simulink model "revised_model"  (R2017a)
settings: Solver=FixedStepAuto  StartTime=0.0  StopTime=60  FixedStep=0.001  RelTol=1e-3
values from neighbouring files (symbols this model uses):
  A = 0    [model_parameter.m]
  a = 0.4    [model_parameter.m]
  a_d = a * negative_gain    (= 0.38)    [model_parameter.m]
  alpha1 = 0.5    [model_parameter.m]
  alpha2 = 0.25    [model_parameter.m]
  B = 1    [model_parameter.m]
  b = 0.4    [model_parameter.m]
  b_d = b * positive_gain    (= 0.42)    [model_parameter.m]
  beta1 = 100    [model_parameter.m]
  beta2 = 300    [model_parameter.m]
  beta3 = 1000    [model_parameter.m]
  C = 1    [model_parameter.m]
  cl = c    (= 0.271)    [model_parameter.m]
  cl_d = c * negative_gain    (= 0.25745)    [model_parameter.m]
  cr = c    (= 0.271)    [model_parameter.m]
  cr_d = c * positive_gain    (= 0.28455)    [model_parameter.m]
  D = 0    [model_parameter.m]
  delta = 0.002    [model_parameter.m]
  k1 = 5    [model_parameter.m]
  k2 = 8    [model_parameter.m]
  k3 = 8    [model_parameter.m]
  k4 = [35 35]    [model_parameter.m]
  k5 = 0    [model_parameter.m]
  k6 = [0.1 0.1]    [model_parameter.m]
  kp = 0.2    [model_parameter.m]
  M = [m 0 0; 0 m 0; 0 0 I]    [model_parameter.m]
  m = 20    [model_parameter.m]
  M_d = [m_d 0 0; 0 m_d 0; 0 0 I_d]    [model_parameter.m]
  m_d = m * positive_gain    (= 21)    [model_parameter.m]
  r = 0.112    [model_parameter.m]
  r_d = r * negative_gain    (= 0.1064)    [model_parameter.m]
  Ts = 0.01    [model_parameter.m]
  ux = 0.02    [model_parameter.m]
  uy = 0.1    [model_parameter.m]
  XICR = 0    [model_parameter.m]
  XICR_d = XICR    (= 0)    [model_parameter.m]
undefined symbols (not defined in the file or in its folder): Continuous, DiscIntNeverNeededParam, Time
libraries: simulink x18, ctrlSharedLib x1
settings Model: Creator=Totorowithme  LastModifiedBy=Totorowithme
settings OptimizationCC: LifeSpan=inf
settings DebuggingCC: SFExecutionAtInitializationDiag=none

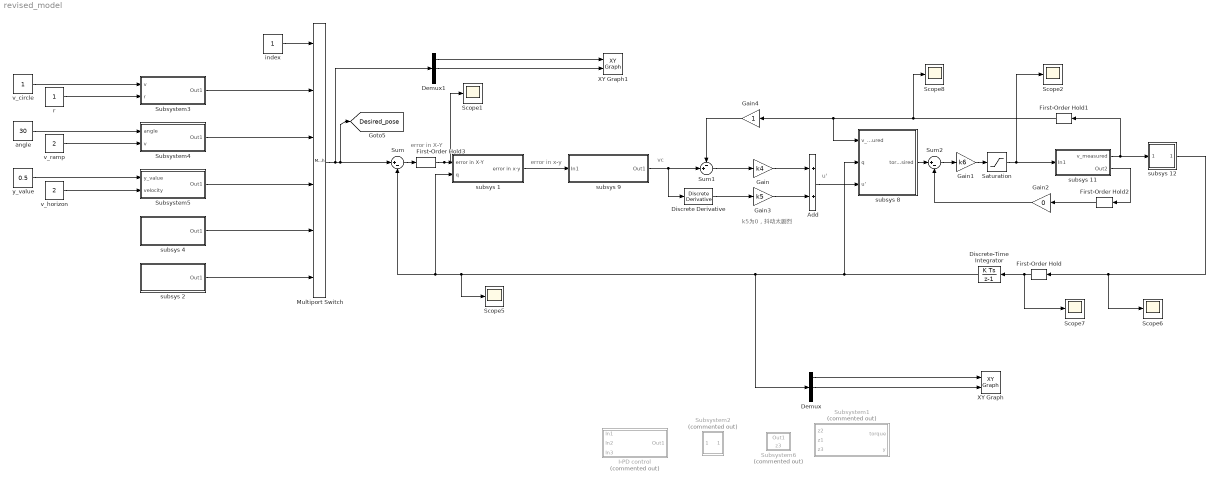
== system revised_model ==
  note: k5为0，抖动太剧烈
  note: u'
  note: vc
  note: error in x-y
  note: error in X-Y
  Add : Sum
  Demux : Demux  Outputs=3
  Demux1 : Demux  Outputs=3
  Discrete Derivative : simulink/Discrete/Discrete Derivative  gainval=1.0  ICPrevScaledInput=0.0  OutMin=[]  OutMax=[]  OutDataType=fixdt(1, 16)  OutScaling=2^-10  DoSatur=off
  Discrete-Time Integrator : DiscreteIntegrator  InitialConditionSetting=State (most efficient)  SampleTime=0.01  ICPrevOutput=DiscIntNeverNeededParam  ICPrevScaledInput=DiscIntNeverNeededParam
  First-Order Hold{,1..3} (4 alike) : simulink/Discrete/First-Order Hold  DisableCoverage=on  Ts=0.01
      settings: SourceProductName=Simulink  SourceProductBaseCode=SL
  Gain : Gain  Gain=k4
  Gain1 : Gain  Gain=k6
  Gain2 : Gain  Gain=0
  Gain3 : Gain  Gain=k5
  Gain4 : Gain
  I-PD control : Subsystem  Commented=on
  Multiport Switch : MultiPortSwitch  Inputs=5
  Saturation : Saturate  UpperLimit=3  LowerLimit=-3
  Scope{1..2,5..8} (6 alike) : Scope
  Subsystem1 : Subsystem  Commented=on
      mask Display: disp('Extended state observer','texmode','on')
  Subsystem2 : Subsystem  Commented=on
      mask Display: disp('inv(S)', 'texmode', 'on')
  Subsystem3 : Subsystem
      mask Display: disp('circle','texmode','on')
  Subsystem4 : Subsystem
      mask Display: disp('ramp','texmode','on')
  Subsystem5 : Subsystem
      mask Display: disp('horizontal line','texmode','on')
  Subsystem6 : Subsystem  Commented=on
      mask Display: disp('inv(H)', 'texmode', 'on')
  Sum : Sum  Inputs=|+-
  Sum1 : Sum  Inputs=-+|
  Sum2 : Sum  Inputs=|+-
  XY Graph : simulink/Sinks/XY Graph  xmin=-12  xmax=12  ymin=-12  ymax=12  st=-1
  XY Graph1 : simulink/Sinks/XY Graph  xmin=-12  xmax=12  ymin=-12  ymax=12  st=-1
  angle : Constant  Value=30
  index : Constant
  r : Constant
  subsys 1 : Subsystem
      mask Display: disp('Transfer from X-Y to x-y','texmode','on')
  subsys 11 : Subsystem
      mask Display: disp('Dynamic function','texmode','on')
  subsys 12 : Subsystem
      mask Display: disp('S(q)','texmode','on')
  subsys 2 : Subsystem
      mask Display: disp('Desired pose','texmode','on')
  subsys 4 : Subsystem
      mask Display: disp('Desired pose','texmode','on')
  subsys 8 : Subsystem
      mask Display: disp('Torque control','texmode','on')
  subsys 9 : Subsystem
      mask Display: disp('Auxiliary velocity control','texmode','on')
  v_circle : Constant
  v_horizon : Constant  Value=2
  v_ramp : Constant  Value=2
  y_value : Constant  Value=0.5
  tag scope: Desired_pose=global
  wires:
  v_circle/1 -> Subsystem3/1(v)
  Subsystem3/1(Out1) -> Multiport Switch/2
  subsys 2/1(Out1) -> Multiport Switch/6
  Subsystem5/1(Out1) -> Multiport Switch/4
  Subsystem4/1(Out1) -> Multiport Switch/3
  r/1 -> Subsystem3/2(r)
  angle/1 -> Subsystem4/1(angle)
  index/1 -> Multiport Switch/1
  v_ramp/1 -> Subsystem4/2(v)
  v_horizon/1 -> Subsystem5/2(velocity)
  subsys 4/1(Out1) -> Multiport Switch/5
  y_value/1 -> Subsystem5/1(y_value)
  Sum/1 -> First-Order Hold3/1
  subsys 1/1(error in x-y) -> subsys 9/1(In1)
  subsys 9/1(Out1) -> Sum1/2, Discrete Derivative/1
  Sum1/1 -> Gain/1
  subsys 12/1(Out1) -> Scope6/1, First-Order Hold/1
  Discrete-Time Integrator/1 -> subsys 8/2(q), Demux/1, Scope5/1, subsys 1/2(q), Sum/2
  Demux/1 -> XY Graph/1
  Demux/2 -> XY Graph/2
  Add/1 -> subsys 8/3(u')
  subsys 11/2(Out2) -> First-Order Hold2/1
  subsys 8/1(torque_desired) -> Sum2/1
  Sum2/1 -> Gain1/1
  Gain1/1 -> Saturation/1
  Discrete Derivative/1 -> Gain3/1
  Gain3/1 -> Add/2
  First-Order Hold/1 -> Discrete-Time Integrator/1, Scope7/1
  First-Order Hold3/1 -> Scope1/1, subsys 1/1(error in X-Y)
  subsys 11/1(v_measured) -> subsys 12/1(In1), First-Order Hold1/1
  Gain4/1 -> Sum1/1
  First-Order Hold2/1 -> Gain2/1
  Gain2/1 -> Sum2/2
  Saturation/1 -> subsys 11/1(In1), Scope2/1
  First-Order Hold1/1 -> Gain4/1, subsys 8/1(v_measured), Scope8/1
  Gain/1 -> Add/1
  Demux1/2 -> XY Graph1/2
  Demux1/1 -> XY Graph1/1
  Multiport Switch/1 -> Sum/1, [Desired_pose], Demux1/1

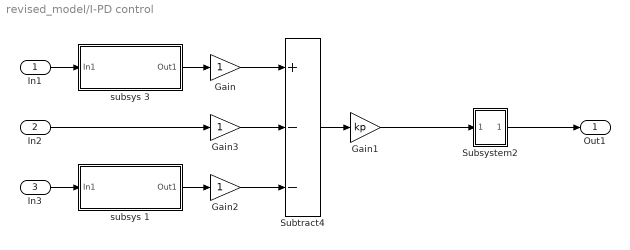
== system revised_model/I-PD control ==
  In1 : Inport
  In2 : Inport  Port=2
  In3 : Inport  Port=3
  Gain : Gain
  Gain1 : Gain  Gain=kp
  Gain2 : Gain
  Gain3 : Gain
  Subsystem2 : Subsystem
      mask Display: disp('inv(S)', 'texmode', 'on')
  Subtract4 : Sum  Inputs=+--
  subsys 1 : Subsystem
      mask Display: disp('transfer2','texmode','on')
  subsys 3 : Subsystem
      mask Display: disp('transfer1','texmode','on')
  Out1 : Outport
  wires:
  In1/1 -> subsys 3/1(In1)
  In3/1 -> subsys 1/1(In1)
  In2/1 -> Gain3/1
  subsys 1/1(Out1) -> Gain2/1
  Subtract4/1 -> Gain1/1
  Gain1/1 -> Subsystem2/1(dq)
  Subsystem2/1(Out1) -> Out1/1
  subsys 3/1(Out1) -> Gain/1
  Gain/1 -> Subtract4/1
  Gain2/1 -> Subtract4/3
  Gain3/1 -> Subtract4/2

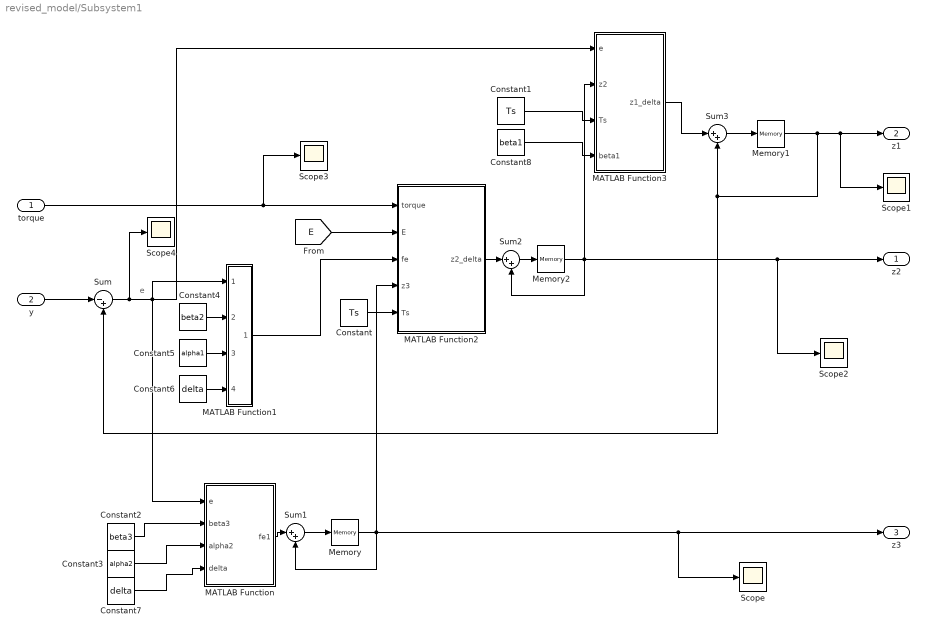
== system revised_model/Subsystem1 ==
  note: e
  torque : Inport
  y : Inport  Port=2
  Constant : Constant  Value=Ts
  Constant1 : Constant  Value=Ts
  Constant2 : Constant  Value=beta3
  Constant3 : Constant  Value=alpha2
  Constant4 : Constant  Value=beta2
  Constant5 : Constant  Value=alpha1
  Constant6 : Constant  Value=delta
  Constant7 : Constant  Value=delta
  Constant8 : Constant  Value=beta1
  MATLAB Function : MATLAB Function  TreatAsAtomicUnit=on
  MATLAB Function1 : MATLAB Function  TreatAsAtomicUnit=on
  MATLAB Function2 : MATLAB Function  TreatAsAtomicUnit=on
  MATLAB Function3 : MATLAB Function  TreatAsAtomicUnit=on
  Memory : Memory  X0=[0 0 0]
  Memory1 : Memory  X0=[0 0 0]
  Memory2 : Memory  X0=[0 0 0]
  Scope{,1..4} (5 alike) : Scope
  Sum : Sum  Inputs=|-+
  Sum1 : Sum  Inputs=|++
  Sum2 : Sum  Inputs=|++
  Sum3 : Sum  Inputs=|++
  z2 : Outport
  z1 : Outport  Port=2
  z3 : Outport  Port=3
  wires:
  y/1 -> Sum/1
  Sum/1 -> Scope4/1, MATLAB Function1/1(e), MATLAB Function3/1(e), MATLAB Function/1(e)
  Sum1/1 -> Memory/1
  MATLAB Function/1(fe1) -> Sum1/1
  MATLAB Function1/1(fe) -> MATLAB Function2/3(fe)
  [E] -> MATLAB Function2/2(E)
  torque/1 -> Scope3/1, MATLAB Function2/1(torque)
  MATLAB Function2/1(z2_delta) -> Sum2/1
  MATLAB Function3/1(z1_delta) -> Sum3/1
  Constant/1 -> MATLAB Function2/5(Ts)
  Constant1/1 -> MATLAB Function3/3(Ts)
  Constant2/1 -> MATLAB Function/2(beta3)
  Constant3/1 -> MATLAB Function/3(alpha2)
  Constant4/1 -> MATLAB Function1/2(beta2)
  Constant5/1 -> MATLAB Function1/3(alpha1)
  Constant6/1 -> MATLAB Function1/4(delta)
  Constant7/1 -> MATLAB Function/4(delta)
  Constant8/1 -> MATLAB Function3/4(beta1)
  Sum2/1 -> Memory2/1
  Sum3/1 -> Memory1/1
  Memory/1 -> Sum1/2, Scope/1, z3/1, MATLAB Function2/4(z3)
  Memory2/1 -> Scope2/1, z2/1, Sum2/2, MATLAB Function3/2(z2)
  Memory1/1 -> Scope1/1, z1/1, Sum3/2, Sum/2

== system revised_model/Subsystem2 ==
  dq : Inport
  MATLAB Function : MATLAB Function  TreatAsAtomicUnit=on
  Out1 : Outport
  wires:
  [S] -> MATLAB Function/1(S)
  dq/1 -> MATLAB Function/2(dq)
  MATLAB Function/1(v) -> Out1/1

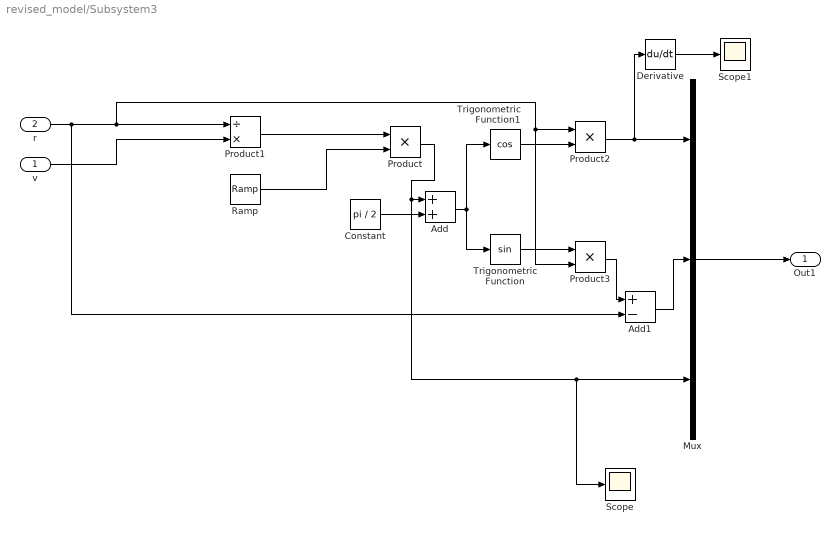
== system revised_model/Subsystem3 ==
  v : Inport
  r : Inport  Port=2
  Add : Sum
  Add1 : Sum  Inputs=+-
  Constant : Constant  Value=pi / 2
  Derivative : Derivative
  Mux : Mux  Inputs=3
  Product : Product
  Product1 : Product  Inputs=/*
  Product2 : Product
  Product3 : Product
  Ramp : simulink/Sources/Ramp  slope=-1  start=0  X0=0
  Scope : Scope
  Scope1 : Scope
  Trigonometric Function : Trigonometry
  Trigonometric Function1 : Trigonometry  Operator=cos
  Out1 : Outport
  wires:
  v/1 -> Product1/2
  r/1 -> Add1/2, Product3/2, Product2/1, Product1/1
  Product1/1 -> Product/1
  Trigonometric Function1/1 -> Product2/2
  Trigonometric Function/1 -> Product3/1
  Product2/1 -> Derivative/1, Mux/1
  Product/1 -> Scope/1, Mux/3, Add/1
  Constant/1 -> Add/2
  Add/1 -> Trigonometric Function/1, Trigonometric Function1/1
  Product3/1 -> Add1/1
  Add1/1 -> Mux/2
  Ramp/1 -> Product/2
  Mux/1 -> Out1/1
  Derivative/1 -> Scope1/1

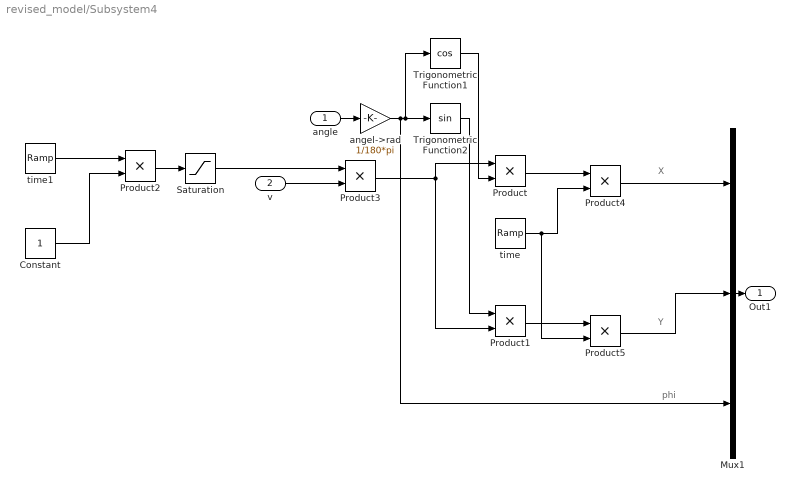
== system revised_model/Subsystem4 ==
  note: phi
  note: Y
  note: X
  angle : Inport
  v : Inport  Port=2
  Constant : Constant
  Mux1 : Mux  Inputs=3
  Product{,1..5} (6 alike) : Product
  Saturation : Saturate  UpperLimit=1  LowerLimit=0
  Trigonometric Function1 : Trigonometry  Operator=cos
  Trigonometric Function2 : Trigonometry
  angel->rad : Gain  Gain=1/180*pi
  time : simulink/Sources/Ramp  slope=1  start=0  X0=0
  time1 : simulink/Sources/Ramp  slope=1  start=0  X0=0
  Out1 : Outport
  wires:
  angle/1 -> angel->rad/1
  Trigonometric Function1/1 -> Product/2
  angel->rad/1 -> Mux1/3, Trigonometric Function1/1, Trigonometric Function2/1
  Trigonometric Function2/1 -> Product1/1
  Product/1 -> Product4/1
  time/1 -> Product5/2, Product4/2
  Product1/1 -> Product5/1
  Product4/1 -> Mux1/1
  Mux1/1 -> Out1/1
  Product5/1 -> Mux1/2
  time1/1 -> Product2/1
  Constant/1 -> Product2/2
  Saturation/1 -> Product3/1
  v/1 -> Product3/2
  Product2/1 -> Saturation/1
  Product3/1 -> Product1/2, Product/1

== system revised_model/Subsystem5 ==
  y_value : Inport
  velocity : Inport  Port=2
  Constant2 : Constant  Value=0
  Mux1 : Mux  Inputs=3
  Product : Product
  time : simulink/Sources/Ramp  slope=1  start=0  X0=0
  Out1 : Outport
  wires:
  y_value/1 -> Mux1/2
  Mux1/1 -> Out1/1
  Constant2/1 -> Mux1/3
  time/1 -> Product/1
  velocity/1 -> Product/2
  Product/1 -> Mux1/1

== system revised_model/Subsystem6 ==
  z3 : Inport
  Constant : Constant  Value=M
  MATLAB Function : MATLAB Function  TreatAsAtomicUnit=on
  Out1 : Outport
  wires:
  [S] -> MATLAB Function/1(S)
  [E] -> MATLAB Function/2(B)
  z3/1 -> MATLAB Function/3(z3)
  MATLAB Function/1(torque_feedback) -> Out1/1
  Constant/1 -> MATLAB Function/4(M)

== system revised_model/subsys 1 ==
  note: 计算 变换矩阵T 参见公式14
  error in X-Y : Inport
  q : Inport  Port=2
  MATLAB Function : MATLAB Function  TreatAsAtomicUnit=on
  Selector : Selector  InputPortWidth=3  IndexOptions=Index vector (dialog)  Indices=[3]  OutputSizes=1
  error in x-y : Outport
  wires:
  error in X-Y/1 -> MATLAB Function/2(error_in_X_Y)
  q/1 -> Selector/1
  Selector/1 -> MATLAB Function/1(phi)
  MATLAB Function/1(error_in_x_y) -> error in x-y/1

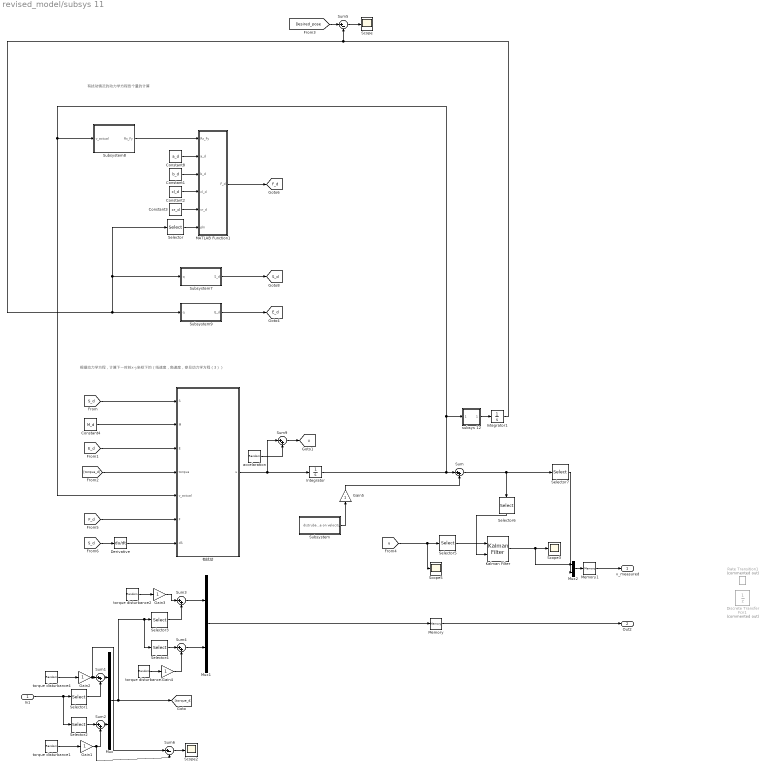
== system revised_model/subsys 11 ==
  note: 根据动力学方程，计算下一时刻x-y坐标下的（线速度，角速度，参见动力学方程（3））
  note: 有扰动情况的动力学方程各个量的计算
  In1 : Inport
  Constant1 : Constant  Value=b_d
  Constant2 : Constant  Value=cl_d
  Constant3 : Constant  Value=cr_d
  Constant4 : Constant  Value=M_d
  Constant8 : Constant  Value=a_d
  Derivative : Derivative
  Discrete Transfer Fcn1 : DiscreteTransferFcn  Commented=on  Denominator=[1 0]  SampleTime=0.01
  Gain{1..5} (5 alike) : Gain
  Integrator : Integrator  InitialCondition=[0 0]
  Integrator1 : Integrator
  Kalman Filter : ctrlSharedLib/Kalman Filter  TimeDomain=Continuous-Time  UseCurrentEstimator=on  ModelSource=Individual A, B, C, D matrices  ModelSourceVariable=ss(0.95,1,1,0,1)  A=A  B=B  C=C  D=D  NumberOfStates=1  NumberOfInputs=1  NumberOfOutputs=1  InitialEstimateSource=Dialog  X0=0  P0=10  UseK=off  UseGH=off  NumberOfProcessNoiseInputs=1  G=1  TimeInvariantG=on  H=0  TimeInvariantH=on  Q=0.0016  TimeInvariantQ=on  R=0.0032  TimeInvariantR=on  N=0  TimeInvariantN=on  AddInputPort=on  AddEnablePort=off  ExternalReset=none  OutputEstimatedY=off  OutputP=off  Ts=0.01
  MATLAB Function1 : MATLAB Function  TreatAsAtomicUnit=on
  Memory : Memory
  Memory1 : Memory  X0=[0 0]
  Mux : Mux  Inputs=2
  Mux1 : Mux  Inputs=2
  Mux2 : Mux  Inputs=2
  Rate Transition1 : RateTransition  Commented=on  OutPortSampleTime=0.01
  Scope{,2..3,5} (4 alike) : Scope
  Selector : Selector  InputPortWidth=3  IndexOptions=Index vector (dialog)  Indices=[3]  OutputSizes=1
  Selector{1,3,5..6} (4 alike) : Selector  InputPortWidth=2  IndexOptions=Index vector (dialog)  Indices=[1]  OutputSizes=1
  Selector2 : Selector  InputPortWidth=2  IndexOptions=Index vector (dialog)  Indices=[2]  OutputSizes=1
  Selector4 : Selector  InputPortWidth=2  IndexOptions=Index vector (dialog)  Indices=[2]  OutputSizes=1
  Selector7 : Selector  InputPortWidth=2  IndexOptions=Index vector (dialog)  Indices=[2]  OutputSizes=1
  Subsystem : Subsystem
  Subsystem7 : Subsystem
  Subsystem8 : Subsystem
  Subsystem9 : Subsystem
  Sum{,1..4,9} (6 alike) : Sum  Inputs=|++
  Sum5 : Sum  Inputs=|+-
  Sum6 : Sum  Inputs=|+-
  accelaration : RandomNumber  Variance=0.0016  Seed=5  SampleTime=0.01
  subsys 12 : Subsystem
      mask Display: disp('S_d(q)','texmode','on')
  torque disturbance1 : RandomNumber  Variance=0.0036  Seed=1  SampleTime=0.01
  torque disturbance2 : RandomNumber  Variance=0.0036  Seed=2  SampleTime=0.01
  torque disturbance3 : RandomNumber  Mean=3  Variance=0.0036  SampleTime=0.01
  torque disturbance4 : RandomNumber  Variance=0.0036  SampleTime=0.01
  有扰动 : MATLAB Function  TreatAsAtomicUnit=on
  v_measured : Outport
  Out2 : Outport  Port=2
  tag scope: E_d=global, F_d=global, S_d=global, u=global
  wires:
  In1/1 -> Selector2/1, Selector1/1
  Selector1/1 -> Sum1/2
  Selector2/1 -> Sum2/1
  torque disturbance1/1 -> Gain1/1
  Sum1/1 -> Mux/1
  Sum2/1 -> Mux/2
  Mux/1 -> Selector4/1, Selector3/1, [torque_d]
  Selector3/1 -> Sum3/2
  Selector4/1 -> Sum4/1
  Sum4/1 -> Mux1/2
  Sum3/1 -> Mux1/1
  torque disturbance3/1 -> Gain4/1
  Gain1/1 -> Sum6/2, Sum2/2
  torque disturbance4/1 -> Gain2/1
  Gain2/1 -> Sum6/1, Sum1/1
  torque disturbance2/1 -> Gain3/1
  Gain3/1 -> Sum3/1
  Gain4/1 -> Sum4/2
  [S_d] -> 有扰动/1(S)
  Constant4/1 -> 有扰动/2(M)
  [E_d] -> 有扰动/3(E)
  [torque_d] -> 有扰动/4(torque)
  [F_d] -> 有扰动/6(F)
  [S_d] -> Derivative/1
  Derivative/1 -> 有扰动/7(dS)
  Subsystem7/1(S_d) -> [S_d]
  Subsystem8/1(Rx_Fy) -> MATLAB Function1/1(Rx_Fy)
  Constant8/1 -> MATLAB Function1/2(a_d)
  Constant1/1 -> MATLAB Function1/3(b_d)
  Constant2/1 -> MATLAB Function1/4(cl_d)
  Selector/1 -> MATLAB Function1/6(phi)
  MATLAB Function1/1(F_d) -> [F_d]
  Subsystem9/1(E_d) -> [E_d]
  Integrator/1 -> Sum/1, subsys 12/1(In1), Subsystem8/1("v_actual "), 有扰动/5(v_actual)
  Constant3/1 -> MATLAB Function1/5(cr_d)
  Integrator1/1 -> Sum5/2, Subsystem7/1(q), Selector/1, Subsystem9/1(q)
  Subsystem/1(distrubance on velocity) -> Gain5/1
  Mux1/1 -> Memory/1
  Gain5/1 -> Sum/2
  Memory/1 -> Out2/1
  subsys 12/1(Out1) -> Integrator1/1
  [Desired_pose] -> Sum5/1
  Sum5/1 -> Scope/1
  Sum6/1 -> Scope2/1
  Kalman Filter/1 -> Mux2/1, Scope3/1
  有扰动/1(u) -> Sum9/1, Integrator/1
  Sum/1 -> Selector6/1, Selector7/1
  [u] -> Scope5/1, Selector5/1
  Selector7/1 -> Mux2/2
  Mux2/1 -> Memory1/1
  Memory1/1 -> v_measured/1
  accelaration/1 -> Sum9/2
  Sum9/1 -> [u]
  Selector6/1 -> Kalman Filter/2
  Selector5/1 -> Kalman Filter/1

== system revised_model/subsys 12 ==
  In1 : Inport
  Product : Product  Multiplication=Matrix(*)
  Out1 : Outport
  wires:
  In1/1 -> Product/2
  [S] -> Product/1
  Product/1 -> Out1/1

== system revised_model/subsys 2 ==
  Clock : Clock
  MATLAB Function : MATLAB Function  TreatAsAtomicUnit=on
  Out1 : Outport
  wires:
  MATLAB Function/1(q) -> Out1/1
  Clock/1 -> MATLAB Function/1(t)

== system revised_model/subsys 4 ==
  Clock : Clock
  MATLAB Function : MATLAB Function  TreatAsAtomicUnit=on
  Out1 : Outport
  wires:
  MATLAB Function/1(q) -> Out1/1
  Clock/1 -> MATLAB Function/1(t)

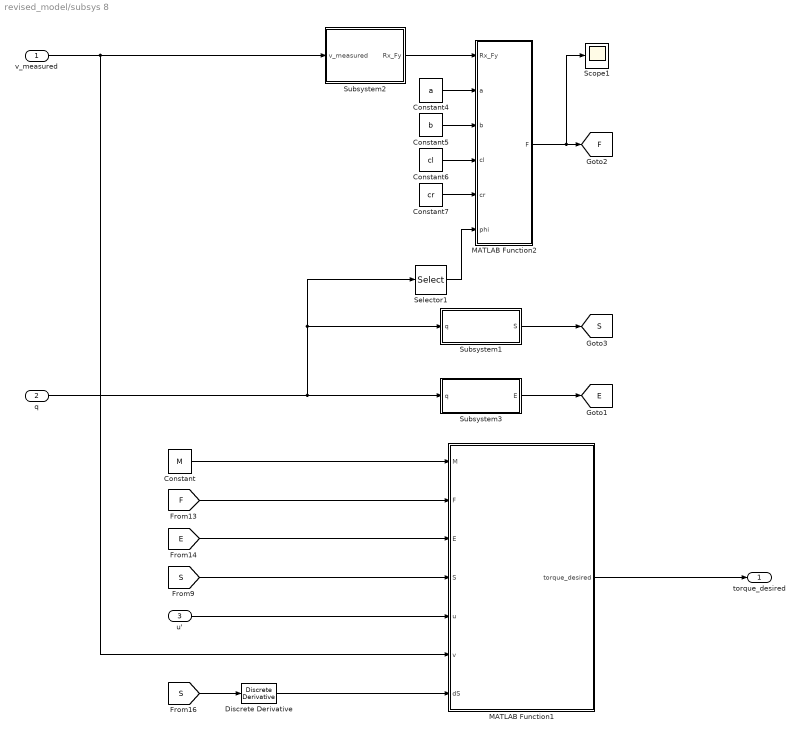
== system revised_model/subsys 8 ==
  v_measured : Inport
  q : Inport  Port=2
  u' : Inport  Port=3
  Constant : Constant  Value=M
  Constant4 : Constant  Value=a
  Constant5 : Constant  Value=b
  Constant6 : Constant  Value=cl
  Constant7 : Constant  Value=cr
  Discrete Derivative : simulink/Discrete/Discrete Derivative  gainval=1.0  ICPrevScaledInput=0.0  OutMin=[]  OutMax=[]  OutDataType=fixdt(1, 16)  OutScaling=2^-10  DoSatur=off
  MATLAB Function1 : MATLAB Function  TreatAsAtomicUnit=on
  MATLAB Function2 : MATLAB Function  TreatAsAtomicUnit=on
  Scope1 : Scope
  Selector1 : Selector  InputPortWidth=3  IndexOptions=Index vector (dialog)  Indices=[3]  OutputSizes=1
  Subsystem1 : Subsystem
  Subsystem2 : Subsystem
  Subsystem3 : Subsystem
  torque_desired : Outport
  tag scope: E=global, F=global, S=global
  wires:
  v_measured/1 -> Subsystem2/1(v_measured), MATLAB Function1/6(v)
  [S] -> Discrete Derivative/1
  Discrete Derivative/1 -> MATLAB Function1/7(dS)
  u'/1 -> MATLAB Function1/5(u)
  [S] -> MATLAB Function1/4(S)
  [E] -> MATLAB Function1/3(E)
  [F] -> MATLAB Function1/2(F)
  Constant/1 -> MATLAB Function1/1(M)
  MATLAB Function1/1(torque_desired) -> torque_desired/1
  Selector1/1 -> MATLAB Function2/6(phi)
  Constant7/1 -> MATLAB Function2/5(cr)
  Constant4/1 -> MATLAB Function2/2(a)
  Constant5/1 -> MATLAB Function2/3(b)
  MATLAB Function2/1(F) -> Scope1/1, [F]
  Subsystem3/1(E) -> [E]
  Constant6/1 -> MATLAB Function2/4(cl)
  Subsystem2/1(Rx_Fy) -> MATLAB Function2/1(Rx_Fy)
  q/1 -> Subsystem1/1(q), Selector1/1, Subsystem3/1(q)
  Subsystem1/1(S) -> [S]

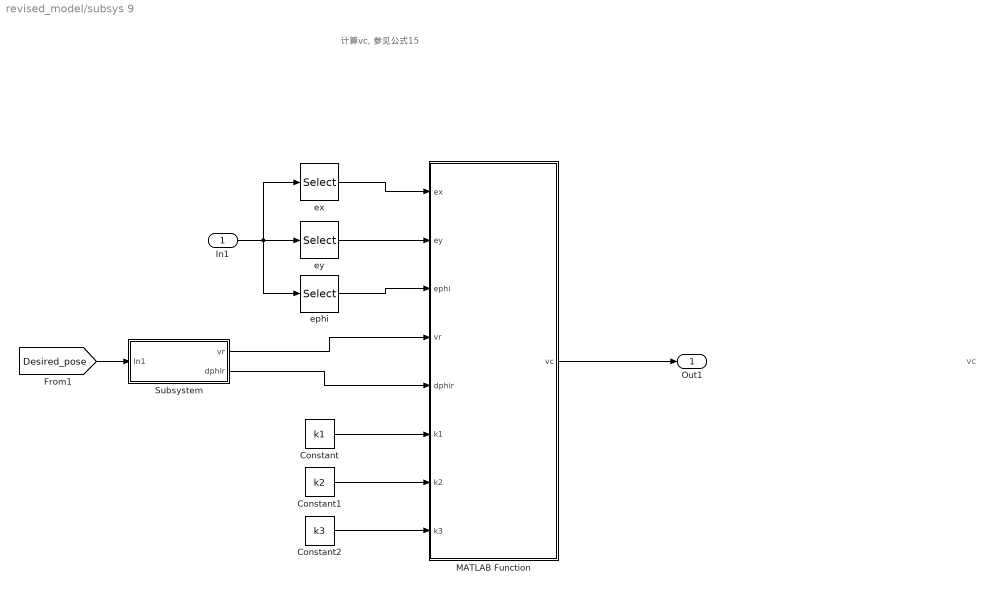
== system revised_model/subsys 9 ==
  note: 计算vc, 参见公式15
  note: vc
  In1 : Inport
  Constant : Constant  Value=k1
  Constant1 : Constant  Value=k2
  Constant2 : Constant  Value=k3
  MATLAB Function : MATLAB Function  TreatAsAtomicUnit=on
  Subsystem : Subsystem
  ephi : Selector  InputPortWidth=3  IndexOptions=Index vector (dialog)  Indices=[3]  OutputSizes=1
  ex : Selector  InputPortWidth=3  IndexOptions=Index vector (dialog)  Indices=[1]  OutputSizes=1
  ey : Selector  InputPortWidth=3  IndexOptions=Index vector (dialog)  Indices=[2]  OutputSizes=1
  Out1 : Outport
  wires:
  In1/1 -> ephi/1, ey/1, ex/1
  [Desired_pose] -> Subsystem/1(In1)
  MATLAB Function/1(vc) -> Out1/1
  ex/1 -> MATLAB Function/1(ex)
  ey/1 -> MATLAB Function/2(ey)
  ephi/1 -> MATLAB Function/3(ephi)
  Subsystem/1(vr) -> MATLAB Function/4(vr)
  Subsystem/2(dphir) -> MATLAB Function/5(dphir)
  Constant/1 -> MATLAB Function/6(k1)
  Constant1/1 -> MATLAB Function/7(k2)
  Constant2/1 -> MATLAB Function/8(k3)

== system revised_model/I-PD control/Subsystem2 ==
  dq : Inport
  MATLAB Function : MATLAB Function  TreatAsAtomicUnit=on
  Out1 : Outport
  wires:
  [S] -> MATLAB Function/1(S)
  dq/1 -> MATLAB Function/2(dq)
  MATLAB Function/1(v) -> Out1/1

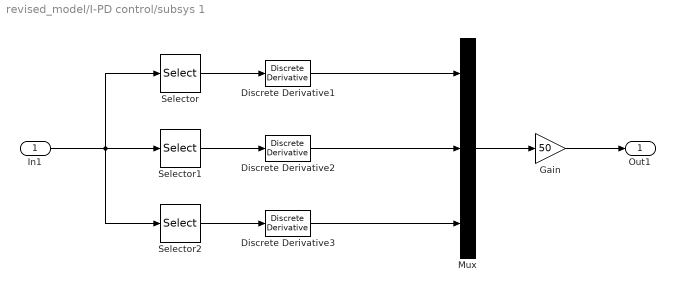
== system revised_model/I-PD control/subsys 1 ==
  In1 : Inport
  Discrete Derivative1 : simulink/Discrete/Discrete Derivative  gainval=1.0  ICPrevScaledInput=0.0  OutMin=[]  OutMax=[]  OutDataType=fixdt(1, 16)  OutScaling=2^-10  DoSatur=off
  Discrete Derivative2 : simulink/Discrete/Discrete Derivative  gainval=1.0  ICPrevScaledInput=0.0  OutMin=[]  OutMax=[]  OutDataType=fixdt(1, 16)  OutScaling=2^-10  DoSatur=off
  Discrete Derivative3 : simulink/Discrete/Discrete Derivative  gainval=1.0  ICPrevScaledInput=0.0  OutMin=[]  OutMax=[]  OutDataType=fixdt(1, 16)  OutScaling=2^-10  DoSatur=off
  Gain : Gain  Gain=50
  Mux : Mux  Inputs=3
  Selector : Selector  InputPortWidth=3  IndexOptions=Index vector (dialog)  Indices=[1]  OutputSizes=1
  Selector1 : Selector  InputPortWidth=3  IndexOptions=Index vector (dialog)  Indices=[2]  OutputSizes=1
  Selector2 : Selector  InputPortWidth=3  IndexOptions=Index vector (dialog)  Indices=[3]  OutputSizes=1
  Out1 : Outport
  wires:
  Selector2/1 -> Discrete Derivative3/1
  Mux/1 -> Gain/1
  In1/1 -> Selector2/1, Selector1/1, Selector/1
  Selector1/1 -> Discrete Derivative2/1
  Selector/1 -> Discrete Derivative1/1
  Discrete Derivative1/1 -> Mux/1
  Discrete Derivative2/1 -> Mux/2
  Discrete Derivative3/1 -> Mux/3
  Gain/1 -> Out1/1

== system revised_model/I-PD control/subsys 3 ==
  In1 : Inport
  Discrete-Time Integrator1 : DiscreteIntegrator  InitialConditionSetting=State (most efficient)  SampleTime=0.01  ICPrevOutput=DiscIntNeverNeededParam  ICPrevScaledInput=DiscIntNeverNeededParam
  Discrete-Time Integrator2 : DiscreteIntegrator  InitialConditionSetting=State (most efficient)  SampleTime=0.01  ICPrevOutput=DiscIntNeverNeededParam  ICPrevScaledInput=DiscIntNeverNeededParam
  Discrete-Time Integrator3 : DiscreteIntegrator  InitialConditionSetting=State (most efficient)  SampleTime=0.01  ICPrevOutput=DiscIntNeverNeededParam  ICPrevScaledInput=DiscIntNeverNeededParam
  Mux : Mux  Inputs=3
  Selector : Selector  InputPortWidth=3  IndexOptions=Index vector (dialog)  Indices=[1]  OutputSizes=1
  Selector1 : Selector  InputPortWidth=3  IndexOptions=Index vector (dialog)  Indices=[2]  OutputSizes=1
  Selector2 : Selector  InputPortWidth=3  IndexOptions=Index vector (dialog)  Indices=[3]  OutputSizes=1
  Out1 : Outport
  wires:
  In1/1 -> Selector2/1, Selector1/1, Selector/1
  Mux/1 -> Out1/1
  Selector/1 -> Discrete-Time Integrator1/1
  Selector1/1 -> Discrete-Time Integrator2/1
  Selector2/1 -> Discrete-Time Integrator3/1
  Discrete-Time Integrator2/1 -> Mux/2
  Discrete-Time Integrator1/1 -> Mux/1
  Discrete-Time Integrator3/1 -> Mux/3

== system revised_model/subsys 11/Subsystem ==
  Gain : Gain  Gain=0
  Gain1 : Gain
  Mux : Mux  Inputs=2
  angular velocity : RandomNumber  Variance=0.0016  Seed=5  SampleTime=0.01
  linear velocity : RandomNumber  Variance=0.0016  Seed=4  SampleTime=0.01
  distrubance on velocity : Outport
  wires:
  linear velocity/1 -> Gain1/1
  angular velocity/1 -> Gain/1
  Mux/1 -> distrubance on velocity/1
  Gain/1 -> Mux/2
  Gain1/1 -> Mux/1

== system revised_model/subsys 11/Subsystem7 ==
  q : Inport
  Constant : Constant  Value=XICR_d
  MATLAB Function : MATLAB Function  TreatAsAtomicUnit=on
  Selector : Selector  InputPortWidth=3  IndexOptions=Index vector (dialog)  Indices=[3]  OutputSizes=1
  S_d : Outport
  wires:
  q/1 -> Selector/1
  Selector/1 -> MATLAB Function/1(phi)
  Constant/1 -> MATLAB Function/2(XICR_d)
  MATLAB Function/1(y) -> S_d/1

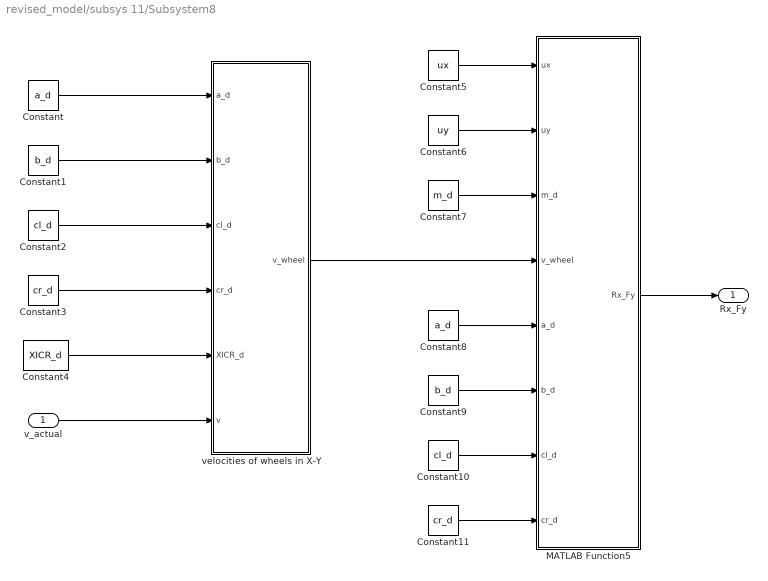
== system revised_model/subsys 11/Subsystem8 ==
  "v_actual " : Inport
  Constant : Constant  Value=a_d
  Constant1 : Constant  Value=b_d
  Constant10 : Constant  Value=cl_d
  Constant11 : Constant  Value=cr_d
  Constant2 : Constant  Value=cl_d
  Constant3 : Constant  Value=cr_d
  Constant4 : Constant  Value=XICR_d
  Constant5 : Constant  Value=ux
  Constant6 : Constant  Value=uy
  Constant7 : Constant  Value=m_d
  Constant8 : Constant  Value=a_d
  Constant9 : Constant  Value=b_d
  MATLAB Function5 : MATLAB Function  TreatAsAtomicUnit=on
  velocities of wheels in X-Y : MATLAB Function  TreatAsAtomicUnit=on
  Rx_Fy : Outport
  wires:
  Constant/1 -> velocities of wheels in X-Y/1(a_d)
  Constant4/1 -> velocities of wheels in X-Y/5(XICR_d)
  Constant1/1 -> velocities of wheels in X-Y/2(b_d)
  Constant2/1 -> velocities of wheels in X-Y/3(cl_d)
  "v_actual "/1 -> velocities of wheels in X-Y/6(v)
  Constant3/1 -> velocities of wheels in X-Y/4(cr_d)
  velocities of wheels in X-Y/1(v_wheel) -> MATLAB Function5/4(v_wheel)
  MATLAB Function5/1(Rx_Fy) -> Rx_Fy/1
  Constant5/1 -> MATLAB Function5/1(ux)
  Constant6/1 -> MATLAB Function5/2(uy)
  Constant7/1 -> MATLAB Function5/3(m_d)
  Constant9/1 -> MATLAB Function5/6(b_d)
  Constant10/1 -> MATLAB Function5/7(cl_d)
  Constant8/1 -> MATLAB Function5/5(a_d)
  Constant11/1 -> MATLAB Function5/8(cr_d)

== system revised_model/subsys 11/Subsystem9 ==
  q : Inport
  Constant : Constant  Value=cl_d
  Constant1 : Constant  Value=cr_d
  Constant2 : Constant  Value=r_d
  MATLAB Function : MATLAB Function  TreatAsAtomicUnit=on
  Selector : Selector  InputPortWidth=3  IndexOptions=Index vector (dialog)  Indices=[3]  OutputSizes=1
  E_d : Outport
  wires:
  Constant1/1 -> MATLAB Function/3(cr_d)
  MATLAB Function/1(E_d) -> E_d/1
  Constant2/1 -> MATLAB Function/4(r_d)
  q/1 -> Selector/1
  Selector/1 -> MATLAB Function/1(phi)
  Constant/1 -> MATLAB Function/2(cl_d)

== system revised_model/subsys 11/subsys 12 ==
  In1 : Inport
  Product : Product  Multiplication=Matrix(*)
  Out1 : Outport
  wires:
  In1/1 -> Product/2
  [S_d] -> Product/1
  Product/1 -> Out1/1

== system revised_model/subsys 8/Subsystem1 ==
  q : Inport
  Constant : Constant  Value=XICR
  MATLAB Function : MATLAB Function  TreatAsAtomicUnit=on
  Selector : Selector  InputPortWidth=3  IndexOptions=Index vector (dialog)  Indices=[3]  OutputSizes=1
  S : Outport
  wires:
  q/1 -> Selector/1
  Selector/1 -> MATLAB Function/1(phi)
  Constant/1 -> MATLAB Function/2(XICR)
  MATLAB Function/1(S) -> S/1

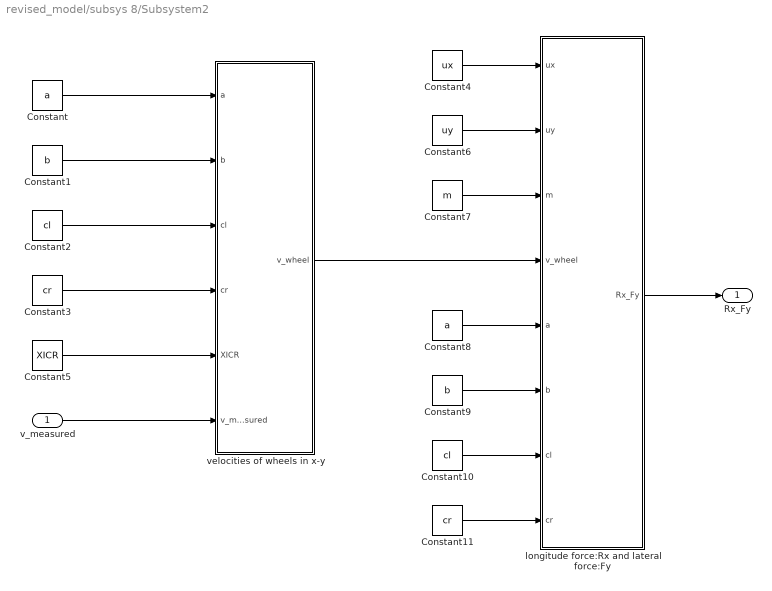
== system revised_model/subsys 8/Subsystem2 ==
  v_measured : Inport
  Constant : Constant  Value=a
  Constant1 : Constant  Value=b
  Constant10 : Constant  Value=cl
  Constant11 : Constant  Value=cr
  Constant2 : Constant  Value=cl
  Constant3 : Constant  Value=cr
  Constant4 : Constant  Value=ux
  Constant5 : Constant  Value=XICR
  Constant6 : Constant  Value=uy
  Constant7 : Constant  Value=m
  Constant8 : Constant  Value=a
  Constant9 : Constant  Value=b
  longitude force:Rx and lateral force:Fy : MATLAB Function  TreatAsAtomicUnit=on
  velocities of wheels in x-y : MATLAB Function  TreatAsAtomicUnit=on
  Rx_Fy : Outport
  wires:
  Constant/1 -> velocities of wheels in x-y/1(a)
  Constant5/1 -> velocities of wheels in x-y/5(XICR)
  Constant1/1 -> velocities of wheels in x-y/2(b)
  Constant2/1 -> velocities of wheels in x-y/3(cl)
  v_measured/1 -> velocities of wheels in x-y/6(v_measured)
  Constant3/1 -> velocities of wheels in x-y/4(cr)
  velocities of wheels in x-y/1(v_wheel) -> longitude force:Rx and lateral force:Fy/4(v_wheel)
  longitude force:Rx and lateral force:Fy/1(Rx_Fy) -> Rx_Fy/1
  Constant4/1 -> longitude force:Rx and lateral force:Fy/1(ux)
  Constant6/1 -> longitude force:Rx and lateral force:Fy/2(uy)
  Constant7/1 -> longitude force:Rx and lateral force:Fy/3(m)
  Constant9/1 -> longitude force:Rx and lateral force:Fy/6(b)
  Constant10/1 -> longitude force:Rx and lateral force:Fy/7(cl)
  Constant8/1 -> longitude force:Rx and lateral force:Fy/5(a)
  Constant11/1 -> longitude force:Rx and lateral force:Fy/8(cr)

== system revised_model/subsys 8/Subsystem3 ==
  q : Inport
  Constant : Constant  Value=cl
  Constant1 : Constant  Value=cr
  Constant2 : Constant  Value=r
  MATLAB Function : MATLAB Function  TreatAsAtomicUnit=on
  Selector : Selector  InputPortWidth=3  IndexOptions=Index vector (dialog)  Indices=[3]  OutputSizes=1
  E : Outport
  wires:
  Constant1/1 -> MATLAB Function/3(cr)
  MATLAB Function/1(E) -> E/1
  Constant2/1 -> MATLAB Function/4(r)
  q/1 -> Selector/1
  Selector/1 -> MATLAB Function/1(phi)
  Constant/1 -> MATLAB Function/2(cl)

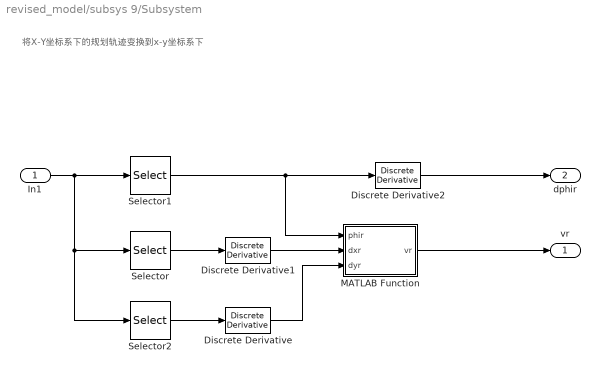
== system revised_model/subsys 9/Subsystem ==
  note: 将X-Y坐标系下的规划轨迹变换到x-y坐标系下
  In1 : Inport
  Discrete Derivative : simulink/Discrete/Discrete Derivative  gainval=1.0  ICPrevScaledInput=0.0  OutMin=[]  OutMax=[]  OutDataType=fixdt(1, 16)  OutScaling=2^-10  DoSatur=off
  Discrete Derivative1 : simulink/Discrete/Discrete Derivative  gainval=1.0  ICPrevScaledInput=0.0  OutMin=[]  OutMax=[]  OutDataType=fixdt(1, 16)  OutScaling=2^-10  DoSatur=off
  Discrete Derivative2 : simulink/Discrete/Discrete Derivative  gainval=1.0  ICPrevScaledInput=0.0  OutMin=[]  OutMax=[]  OutDataType=fixdt(1, 16)  OutScaling=2^-10  DoSatur=off
  MATLAB Function : MATLAB Function  TreatAsAtomicUnit=on
  Selector : Selector  InputPortWidth=3  IndexOptions=Index vector (dialog)  Indices=[1]  OutputSizes=1
  Selector1 : Selector  InputPortWidth=3  IndexOptions=Index vector (dialog)  Indices=[3]  OutputSizes=1
  Selector2 : Selector  InputPortWidth=3  IndexOptions=Index vector (dialog)  Indices=[2]  OutputSizes=1
  vr : Outport
  dphir : Outport  Port=2
  wires:
  In1/1 -> Selector2/1, Selector/1, Selector1/1
  Selector2/1 -> Discrete Derivative/1
  Selector/1 -> Discrete Derivative1/1
  Discrete Derivative1/1 -> MATLAB Function/2(dxr)
  Discrete Derivative/1 -> MATLAB Function/3(dyr)
  Selector1/1 -> Discrete Derivative2/1, MATLAB Function/1(phir)
  MATLAB Function/1(vr) -> vr/1
  Discrete Derivative2/1 -> dphir/1

== matlab function revised_model/subsys 1/MATLAB Function ==
  data: phi input; error_in_x_y output; error_in_X_Y input
function error_in_x_y = fcn(phi, error_in_X_Y)
T = [cos(phi) sin(phi) 0; -sin(phi) cos(phi) 0; 0 0 1];
error_in_x_y = T * error_in_X_Y;

== matlab function revised_model/subsys 9/Subsystem/MATLAB Function ==
  data: phir input; vr output; dxr input; dyr input
function vr = fcn(phir, dxr, dyr)

vr = dxr*cos(phir) + dyr*sin(phir);

== matlab function revised_model/subsys 9/MATLAB Function ==
  data: ex input; vc output; ey input; ephi input; vr input; dphir input; k1 input; k2 input; k3 input
function vc = fcn(ex, ey, ephi, vr, dphir,k1,k2,k3)
y1 = vr*cos(ephi) + k1*ex;
y2 = dphir+k2*vr*ey + k3*vr*sin(ephi);
vc = [y1; y2];

== matlab function revised_model/subsys 8/MATLAB Function1 ==
  data: M input; torque_desired output; F input; E input; S input; u input; v input; dS input
function torque_desired = fcn(M, F, E, S, u, v, dS)
torque_desired = inv(S'*E)*(S'*M*S*u +S'*M*dS*v +S'*F);

== matlab function revised_model/subsys 8/MATLAB Function2 ==
  data: Rx_Fy input; F output; a input; b input; cl input; cr input; phi input
function F = fcn(Rx_Fy,a,b,cl,cr,phi)
Rx = Rx_Fy(1) + Rx_Fy(2) + Rx_Fy(3) + Rx_Fy(4);
Fy = Rx_Fy(5) + Rx_Fy(6) + Rx_Fy(7) + Rx_Fy(8);
Mr = a * (Rx_Fy(5) + Rx_Fy(6)) - b * (Rx_Fy(7) + Rx_Fy(8)) + cr * (Rx_Fy(3) + Rx_Fy(4)) - cl * (Rx_Fy(1) + Rx_Fy(2));
F1 = Rx * cos(phi) - Fy*sin(phi);
F2 = Rx*sin(phi) + Fy*cos(phi);
F = [F1; F2; Mr];

== matlab function revised_model/subsys 11/MATLAB Function1 ==
  data: Rx_Fy input; F_d output; a_d input; b_d input; cl_d input; cr_d input; phi input
function F_d = fcn(Rx_Fy,a_d,b_d,cl_d,cr_d,phi)
Rx = Rx_Fy(1) + Rx_Fy(2) + Rx_Fy(3) + Rx_Fy(4);
Fy = Rx_Fy(5) + Rx_Fy(6) + Rx_Fy(7) + Rx_Fy(8);
Mr = a_d * (Rx_Fy(5) + Rx_Fy(6)) - b_d * (Rx_Fy(7) + Rx_Fy(8)) + cr_d * (Rx_Fy(3) + Rx_Fy(4)) - cl_d * (Rx_Fy(1) + Rx_Fy(2));
F1 = Rx * cos(phi) - Fy*sin(phi);
F2 = Rx*sin(phi) + Fy*cos(phi);
F_d = [F1; F2; Mr];

== matlab function revised_model/subsys 11/Subsystem7/MATLAB Function ==
  data: phi input; y output; XICR_d input
function y = fcn(phi, XICR_d)

y = [cos(phi) XICR_d*sin(phi); sin(phi) -XICR_d*cos(phi); 0 1];

== matlab function revised_model/subsys 11/Subsystem8/MATLAB Function5 ==
  data: ux input; uy input; Rx_Fy output; m_d input; v_wheel input; a_d input; b_d input; cl_d input; cr_d input
function Rx_Fy = fcn(ux, uy, m_d, v_wheel, a_d, b_d, cl_d, cr_d)
sign_wheel = [0 0 0 0];
Rx_Fy = [0 0 0 0 0 0 0 0];
for i = 1:4
v_i = v_wheel(i);
if v_i <= 0.01 && v_i >= -0.01
    sign_wheel(i) = v_i * 100;
else
    sign_wheel(i) = sign(v_i);
end
end
Rx_Fy(1) = sign_wheel(1) * ux * m_d * 9.8 * b_d / (a_d + b_d) * cr_d / (cl_d + cr_d);
Rx_Fy(2) = sign_wheel(1) * ux * m_d * 9.8 * a_d / (a_d + b_d) * cr_d / (cl_d + cr_d);
Rx_Fy(3) = sign_wheel(2) * ux * m_d * 9.8 * b_d / (a_d + b_d) * cl_d / (cl_d + cr_d);
Rx_Fy(4) = sign_wheel(2) * ux * m_d * 9.8 * a_d / (a_d + b_d) * cl_d / (cl_d + cr_d);

Rx_Fy(5) = sign_wheel(3) * uy * m_d * 9.8 * b_d / (a_d + b_d) * cr_d / (cl_d + cr_d);
Rx_Fy(6) = sign_wheel(3) * uy * m_d * 9.8 * b_d / (a_d + b_d) * cl_d / (cl_d + cr_d);
Rx_Fy(7) = sign_wheel(4) * uy * m_d * 9.8 * a_d / (a_d + b_d) * cr_d / (cl_d + cr_d);
Rx_Fy(8) = sign_wheel(4) * uy * m_d * 9.8 * a_d / (a_d + b_d) * cl_d / (cl_d + cr_d);

== matlab function revised_model/subsys 11/Subsystem8/velocities of wheels in X-Y ==
  data: a_d input; v_wheel output; b_d input; cl_d input; cr_d input; XICR_d input; v input
function v_wheel = fcn(a_d,b_d,cl_d,cr_d,XICR_d,v)
y11 = 1;
y12 = -cl_d;
y21 = 1;
y22 = cr_d;
y31 = 0;
y32 = -XICR_d + a_d;
y41 = 0;
y42 = -XICR_d - b_d;
v_wheel = [y11 y12; y21 y22; y31 y32; y41 y42] * v;

== matlab function revised_model/subsys 11/Subsystem9/MATLAB Function ==
  data: phi input; E_d output; cl_d input; cr_d input; r_d input
function E_d = fcn(phi, cl_d, cr_d, r_d)
E11 = cos(phi)/r_d;
E12 = cos(phi)/r_d;
E21 = sin(phi)/r_d;
E22 = sin(phi)/r_d;
E31 = -cl_d/r_d;
E32 = +cr_d/r_d;
E_d = [E11 E12; E21 E22; E31 E32];

== matlab function revised_model/Subsystem1/MATLAB Function ==
  data: e input; fe1 output; beta3 input; alpha2 input; delta input
function fe1 = fcn(e, beta3, alpha2, delta)
fe1 = [0; 0; 0];
for i = 1:3
    if abs(e(i)) <= delta
        fe1(i) = -beta3 * e(i) / delta ^ (alpha2 - 1);
    else
        fe1(i) = -beta3 * abs(e(i)) ^ alpha2 * sign(e(i));
    end
end

== matlab function revised_model/Subsystem1/MATLAB Function1 ==
  data: e input; fe output; beta2 input; alpha1 input; delta input
function fe = fcn(e, beta2, alpha1, delta)
fe = [0; 0; 0];
for i = 1:3
    if abs(e(i)) <= delta
        fe(i) = -beta2 * e(i) / delta ^ (alpha1 - 1);
    else
        fe(i) = -beta2 * abs(e(i)) ^ alpha1 * sign(e(i));
    end
end

== matlab function revised_model/Subsystem1/MATLAB Function2 ==
  data: torque input; z2_delta output; E input; fe input; z3 input; Ts input
function z2_delta = fcn(torque, E, fe, z3, Ts)
z2_delta = Ts .*(z3 + E * torque + fe);

== matlab function revised_model/subsys 8/Subsystem1/MATLAB Function ==
  data: phi input; S output; XICR input
function S = fcn(phi, XICR)

S = [cos(phi) XICR*sin(phi); sin(phi) -XICR*cos(phi); 0 1];

== matlab function revised_model/Subsystem1/MATLAB Function3 ==
  data: e input; z1_delta output; z2 input; Ts input; beta1 input
function z1_delta = fcn(e, z2, Ts, beta1)
z1_delta = Ts .* (z2 - beta1 .* e);

== matlab function revised_model/subsys 4/MATLAB Function ==
  data: t input; q output
function q = fcn(t)
%#codegen
x = 5*sin((t+1/360)*0.2);
y = 5*sin(2*t*0.2);

tf = t - 1e-3;
xf = 5*sin((tf+1/360)*0.2);
yf = 5*sin(2 * tf*0.2);


phi = atan2((y - yf) , (x - xf));
if phi < 0
    phi = (phi + 2*pi);
end

q = [x;y;phi];

== matlab function revised_model/Subsystem6/MATLAB Function ==
  data: S input; torque_feedback output; B input; z3 input; M input
function torque_feedback = fcn(S, B, z3, M)
torque_feedback = pinv(S * pinv(S' * M * S) * S' * B) * z3;

== matlab function revised_model/subsys 8/Subsystem2/velocities of wheels in x-y ==
  data: a input; v_wheel output; b input; cl input; cr input; XICR input; v_measured input
function v_wheel = fcn(a,b,cl,cr,XICR,v_measured)
y11 = 1;
y12 = -cl;
y21 = 1;
y22 = cr;
y31 = 0;
y32 = -XICR + a;
y41 = 0;
y42 = -XICR - b;
v_wheel = [y11 y12; y21 y22; y31 y32; y41 y42] * v_measured;

== matlab function revised_model/subsys 11/有扰动 ==
  data: S input; u output; M input; E input; torque input; v_actual input; F input; dS input
function u = fcn(S,M,E,torque,v_actual,F,dS)

u = pinv(S'*M*S) * S'* (E*torque - M*dS*v_actual - F);

== matlab function revised_model/subsys 2/MATLAB Function ==
  data: t input; q output
function q = fcn(t)
%#codegen
x = 5*sin((t+1/360)*pi);
y = 5*sin(2*t*pi);

tf = t - 1e-3;
xf = 5*sin((tf+1/360)*pi);
yf = 5*sin(2 * tf*pi);


phi = atan2((y - yf) , (x - xf));
if phi < 0
    phi = (phi + 2*pi);
end

q = [x;y;phi];

== matlab function revised_model/Subsystem2/MATLAB Function ==
  data: S input; v output; dq input
function v = fcn(S,dq)
v = pinv(S) * dq;

== matlab function revised_model/I-PD control/Subsystem2/MATLAB Function ==
  data: S input; v output; dq input
function v = fcn(S,dq)
v = pinv(S) * dq;

== matlab function revised_model/subsys 8/Subsystem3/MATLAB Function ==
  data: phi input; E output; cl input; cr input; r input
function E = fcn(phi, cl, cr, r)
E11 = cos(phi)/r;
E12 = cos(phi)/r;
E21 = sin(phi)/r;
E22 = sin(phi)/r;
E31 = -cl/r;
E32 = +cr/r;
E = [E11 E12; E21 E22; E31 E32];

== matlab function revised_model/subsys 8/Subsystem2/longitude force:Rx and lateral force:Fy ==
  data: ux input; uy input; Rx_Fy output; m input; v_wheel input; a input; b input; cl input; cr input
function Rx_Fy = fcn(ux, uy, m, v_wheel, a, b, cl, cr)
sign_wheel = [0 0 0 0];
Rx_Fy = [0 0 0 0 0 0 0 0];
for i = 1:4
v_i = v_wheel(i);
if v_i <= 0.01 && v_i >= -0.01
    sign_wheel(i) = v_i * 100;
else
    sign_wheel(i) = sign(v_i);
end
end
Rx_Fy(1) = sign_wheel(1) * ux * m * 9.8 * b / (a + b) * cr / (cl + cr);
Rx_Fy(2) = sign_wheel(1) * ux * m * 9.8 * a / (a + b) * cr / (cl + cr);
Rx_Fy(3) = sign_wheel(2) * ux * m * 9.8 * b / (a + b) * cl / (cl + cr);
Rx_Fy(4) = sign_wheel(2) * ux * m * 9.8 * a / (a + b) * cl / (cl + cr);

Rx_Fy(5) = sign_wheel(3) * uy * m * 9.8 * b / (a + b) * cr / (cl + cr);
Rx_Fy(6) = sign_wheel(3) * uy * m * 9.8 * b / (a + b) * cl / (cl + cr);
Rx_Fy(7) = sign_wheel(4) * uy * m * 9.8 * a / (a + b) * cr / (cl + cr);
Rx_Fy(8) = sign_wheel(4) * uy * m * 9.8 * a / (a + b) * cl / (cl + cr);
